simulink model "MCU_PWMPrdChg_Merge"  (R2022b)
settings: Solver=VariableStepAuto  StartTime=0.0  StopTime=10.0  RelTol=1e-3
values from neighbouring files (symbols this model uses):
  C_PWMPrdChg_PwmDefLimit_u16 = 0.0    [MCU_PWMPrdChg_Sldd.sldd]    (also in MCU_PWMPrdChg_Sldd_objects.m = myPackage.Parameter)
  C_PWMPrdChg_PwmHighLimit_u16 = 0.0    [MCU_PWMPrdChg_Sldd.sldd]    (also in MCU_PWMPrdChg_Sldd_objects.m = myPackage.Parameter)
  C_PWMPrdChg_PwmLowLimit_u16 = 0.0    [MCU_PWMPrdChg_Sldd.sldd]    (also in MCU_PWMPrdChg_Sldd_objects.m = myPackage.Parameter)
undefined symbols (not defined in the file or in its folder): MAIN_CPU_FRE, ParamCfg_MotorNp_u16, ParamCfg_PwmFreqHigh_u16, ParamCfg_PwmFreqLow_u16, ParamCfg_PwmLowSpeed_u16, ParamCfg_Pwmprdchgen_u16, ParamCfg_PwmPrdChgEn_u16, ParamCfg_RotateNp_u16, PWM_PERIOD_H
libraries: simulink x2
settings Model: DataDictionary=MCU_PWMPrdChg_Sldd.sldd  Creator=ZYH  LastModifiedBy=ZYH
settings RTWCC: CustomHeaderCode="#include \"myfile.h\""  CustomSource=myfile.c

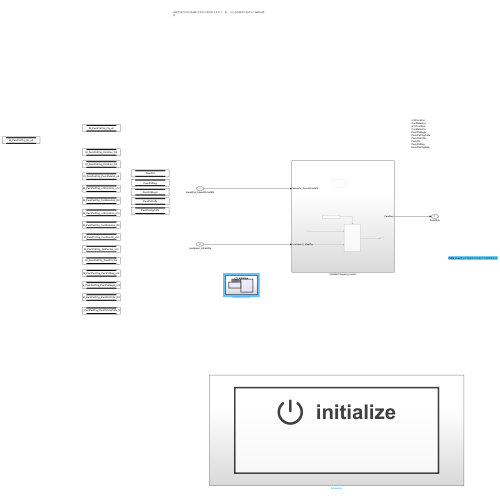
[thumbnail: Simulink's stored preview of the top-level diagram]
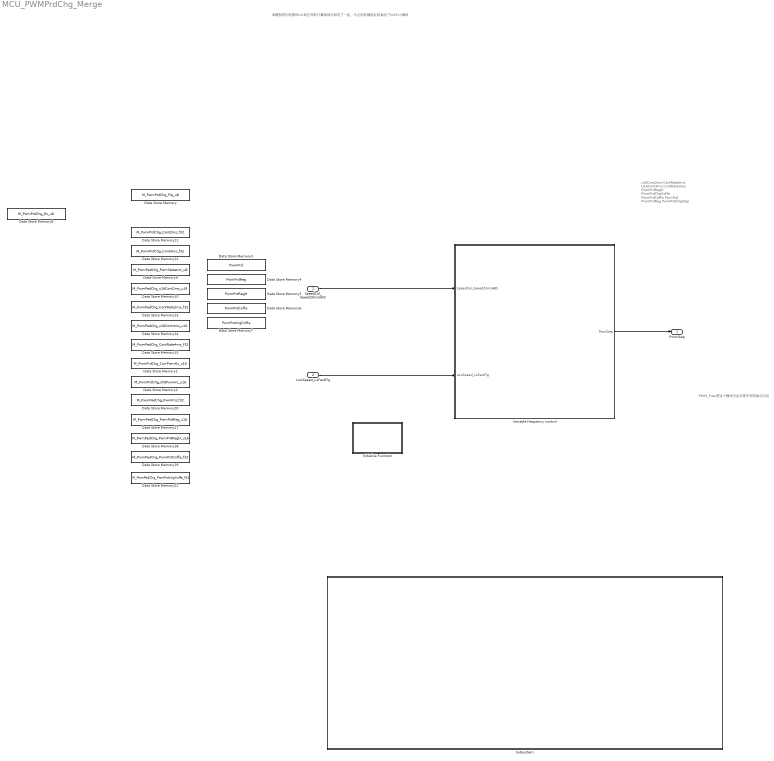
== system MCU_PWMPrdChg_Merge ==
  note: 该模型将代码里的Init和正常的计算两部分和在了一起，与之前的模型比较省去了InitFcn模块
  note: PWM_Freq是这个模块引出还是手写初始化引出
  note: u16Cont2ms
      | ContRate2ms
      | U16Cont4ms
      | ContRate4ms
      | PwmPrdRegH
      | PwmPrdChgCoffe
      | PwmPrdCoffe
      | PwmPrd
      | PwmPrdReg
      | PwmPrdChgStep
  SpeedCal_Speed20msABS : Inport
  LowSpeed_LsFastFlg : Inport  Port=2
  Data Store Memory : DataStoreMemory  DataStoreName=M_PwmPrdChg_Flg_u8  WriteAfterWriteMsg=warning  ShowAdditionalParam=off  OutDataTypeStr=uint8  StateMustResolveToSignalObject=on
  Data Store Memory1 : DataStoreMemory  DataStoreName=M_PwmPrdChg_CurrPwmHz_u16  WriteAfterWriteMsg=warning  ShowAdditionalParam=off  OutDataTypeStr=uint16  StateMustResolveToSignalObject=on
  Data Store Memory10 : DataStoreMemory  DataStoreName=M_PwmPedChg_u16Cont2ms_u16  WriteAfterWriteMsg=warning  ShowAdditionalParam=off  OutDataTypeStr=uint16  StateMustResolveToSignalObject=on
  Data Store Memory11 : DataStoreMemory  DataStoreName=M_PwmPrdChg_Cont2ms_f32  WriteAfterWriteMsg=warning  ShowAdditionalParam=off  OutDataTypeStr=single  StateMustResolveToSignalObject=on
  Data Store Memory12 : DataStoreMemory  DataStoreName=M_PwmPrdChg_Cont4ms_f32  WriteAfterWriteMsg=warning  ShowAdditionalParam=off  OutDataTypeStr=single  StateMustResolveToSignalObject=on
  Data Store Memory13 : DataStoreMemory  DataStoreName=M_PwmPedChg_ContRate2ms_f32  WriteAfterWriteMsg=warning  ShowAdditionalParam=off  OutDataTypeStr=single  StateMustResolveToSignalObject=on
  Data Store Memory14 : DataStoreMemory  DataStoreName=M_PwmPedChg_u16Cont4ms_u16  WriteAfterWriteMsg=warning  ShowAdditionalParam=off  OutDataTypeStr=uint16  StateMustResolveToSignalObject=on
  Data Store Memory15 : DataStoreMemory  DataStoreName=M_PwmPedChg_ContRate4ms_f32  WriteAfterWriteMsg=warning  ShowAdditionalParam=off  OutDataTypeStr=single  StateMustResolveToSignalObject=on
  Data Store Memory17 : DataStoreMemory  DataStoreName=M_PwmPedChg_PwmPrdReg_u16  WriteAfterWriteMsg=warning  ShowAdditionalParam=off  OutDataTypeStr=uint16  StateMustResolveToSignalObject=on
  Data Store Memory18 : DataStoreMemory  DataStoreName=M_PwmPedChg_PwmPrdRegH_u16  WriteAfterWriteMsg=warning  ShowAdditionalParam=off  OutDataTypeStr=uint16  StateMustResolveToSignalObject=on
  Data Store Memory19 : DataStoreMemory  DataStoreName=M_PwmPedChg_PwmPrdCoffe_f32  WriteAfterWriteMsg=warning  ShowAdditionalParam=off  OutDataTypeStr=single  StateMustResolveToSignalObject=on
  Data Store Memory2 : DataStoreMemory  DataStoreName=M_PwmPrdChg_OldPwmHz_u16  WriteAfterWriteMsg=warning  ShowAdditionalParam=off  OutDataTypeStr=uint16  StateMustResolveToSignalObject=on
  Data Store Memory20 : DataStoreMemory  DataStoreName=M_PwmPedChg_PwmPrd_f32  WriteAfterWriteMsg=warning  ShowAdditionalParam=off  OutDataTypeStr=single  StateMustResolveToSignalObject=on
  Data Store Memory21 : DataStoreMemory  DataStoreName=M_PwmPedChg_PwmPrdchgCoffe_f32  WriteAfterWriteMsg=warning  ShowAdditionalParam=off  OutDataTypeStr=single  StateMustResolveToSignalObject=on
  Data Store Memory3 : DataStoreMemory  DataStoreName=PwmPrd  WriteAfterWriteMsg=warning  ShowAdditionalParam=off
  Data Store Memory4 : DataStoreMemory  DataStoreName=PwmPrdReg  WriteAfterWriteMsg=warning  ShowAdditionalParam=off
  Data Store Memory5 : DataStoreMemory  DataStoreName=PwmPrdRegH  WriteAfterWriteMsg=warning  ShowAdditionalParam=off
  Data Store Memory6 : DataStoreMemory  DataStoreName=PwmPrdCoffe  WriteAfterWriteMsg=warning  ShowAdditionalParam=off
  Data Store Memory7 : DataStoreMemory  DataStoreName=PwmPrdchgCoffe  WriteAfterWriteMsg=warning  ShowAdditionalParam=off
  Data Store Memory8 : DataStoreMemory  DataStoreName=M_PwmPrdChg_En_u8  WriteAfterWriteMsg=warning  ShowAdditionalParam=off  OutDataTypeStr=uint8  StateMustResolveToSignalObject=on
  Data Store Memory9 : DataStoreMemory  DataStoreName=M_PwmPedChg_PwmStateInit_u8  WriteAfterWriteMsg=warning  ShowAdditionalParam=off  OutDataTypeStr=uint8  StateMustResolveToSignalObject=on
  Initialize Function : Subsystem  TreatAsAtomicUnit=on
  Subsystem : Subsystem
  Variable frequency control : Subsystem
  PwmStep : Outport
  wires:
  Variable frequency control/1(PwmStep) -> PwmStep/1
  SpeedCal_Speed20msABS/1 -> Variable frequency control/1(SpeedCal_Speed20msABS)
  LowSpeed_LsFastFlg/1 -> Variable frequency control/2(LowSpeed_LsFastFlg)

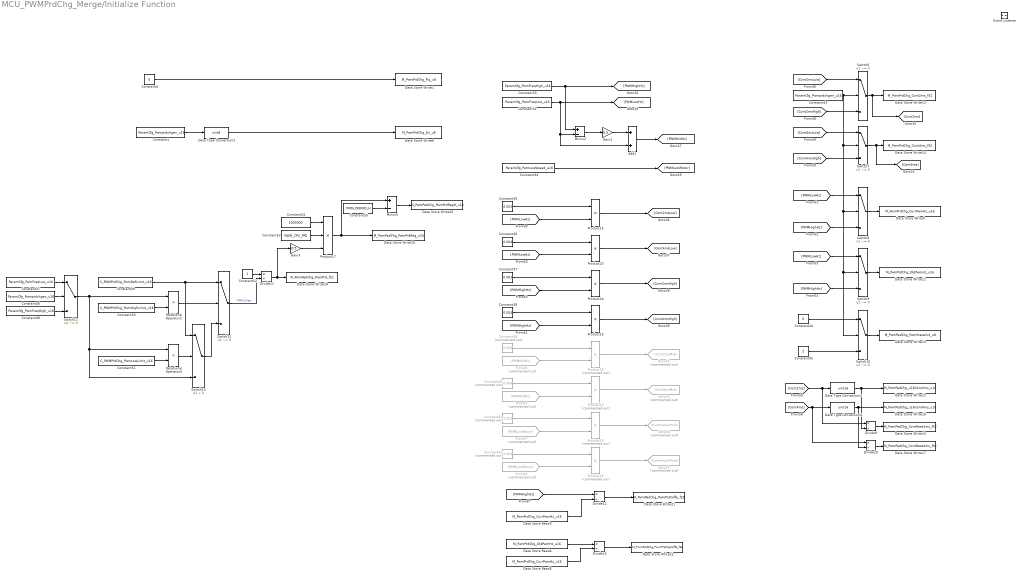
== system MCU_PWMPrdChg_Merge/Initialize Function ==
  Add1 : Sum  OutDataTypeStr=uint16
  Constant1 : Constant  Value=ParamCfg_Pwmprdchgen_u16  OutDataTypeStr=uint16
  Constant32 : Constant  Value=ParamCfg_PwmFreqLow_u16  OutDataTypeStr=uint16
  Constant33 : Constant  Value=ParamCfg_PwmFreqHigh_u16  OutDataTypeStr=uint16
  Constant34 : Constant  Value=ParamCfg_PwmLowSpeed_u16  OutDataTypeStr=uint16
  Constant35 : Constant  Value=0.002  OutDataTypeStr=single
  Constant36 : Constant  Value=0.004  OutDataTypeStr=single
  Constant37 : Constant  Value=0.002  OutDataTypeStr=single
  Constant38 : Constant  Value=0.004  OutDataTypeStr=single
  Constant39 : Constant  Commented=on  Value=0.002  OutDataTypeStr=single
  Constant4 : Constant  Value=0  OutDataTypeStr=uint8
  Constant40 : Constant  Commented=on  Value=0.004  OutDataTypeStr=single
  Constant41 : Constant  Commented=on  Value=0.002  OutDataTypeStr=single
  Constant42 : Constant  Commented=on  Value=0.004  OutDataTypeStr=single
  Constant43 : Constant  Value=ParamCfg_Pwmprdchgen_u16  OutDataTypeStr=uint16
  Constant44 : Constant  Value=0  OutDataTypeStr=uint8
  Constant45 : Constant  Value=2  OutDataTypeStr=uint8
  Constant46 : Constant  Value=ParamCfg_Pwmprdchgen_u16  OutDataTypeStr=uint16
  Constant47 : Constant  Value=ParamCfg_PwmFreqLow_u16  OutDataTypeStr=uint16
  Constant48 : Constant  Value=ParamCfg_PwmFreqHigh_u16  OutDataTypeStr=uint16
  Constant49 : Constant  Value=C_PWMPrdChg_PwmDefLimit_u16  OutDataTypeStr=uint16
  Constant50 : Constant  Value=C_PWMPrdChg_PwmHighLimit_u16  OutDataTypeStr=uint16
  Constant51 : Constant  Value=C_PWMPrdChg_PwmLowLimit_u16  OutDataTypeStr=uint16
  Constant52 : Constant  OutDataTypeStr=single
  Constant53 : Constant  Value=MAIN_CPU_FRE  OutDataTypeStr=uint16
  Constant54 : Constant  Value=1000000  OutDataTypeStr=single
  Constant55 : Constant  Value=PWM_PERIOD_H  OutDataTypeStr=uint16
  Data Store Read3 : DataStoreRead  DataStoreName=M_PwmPrdChg_CurrPwmHz_u16  IndexOptions=Index vector (dialog)  Indices=1  OutputSizes=1
  Data Store Read4 : DataStoreRead  DataStoreName=M_PwmPrdChg_OldPwmHz_u16  IndexOptions=Index vector (dialog)  Indices=1  OutputSizes=1
  Data Store Read5 : DataStoreRead  DataStoreName=M_PwmPrdChg_CurrPwmHz_u16  IndexOptions=Index vector (dialog)  Indices=1  OutputSizes=1
  Data Store Write1 : DataStoreWrite  DataStoreName=M_PwmPrdChg_Flg_u8  IndexOptions=Index vector (dialog)  Indices=1  OutputSizes=1
  Data Store Write10 : DataStoreWrite  DataStoreName=M_PwmPedChg_PwmStateInit_u8  IndexOptions=Index vector (dialog)  Indices=1  OutputSizes=1
  Data Store Write11 : DataStoreWrite  DataStoreName=M_PwmPrdChg_OldPwmHz_u16  IndexOptions=Index vector (dialog)  Indices=1  OutputSizes=1
  Data Store Write12 : DataStoreWrite  DataStoreName=M_PwmPedChg_u16Cont2ms_u16  IndexOptions=Index vector (dialog)  Indices=1  OutputSizes=1
  Data Store Write13 : DataStoreWrite  DataStoreName=M_PwmPrdChg_Cont2ms_f32  IndexOptions=Index vector (dialog)  Indices=1  OutputSizes=1
  Data Store Write14 : DataStoreWrite  DataStoreName=M_PwmPrdChg_Cont4ms_f32  IndexOptions=Index vector (dialog)  Indices=1  OutputSizes=1
  Data Store Write15 : DataStoreWrite  DataStoreName=M_PwmPedChg_ContRate2ms_f32  IndexOptions=Index vector (dialog)  Indices=1  OutputSizes=1
  Data Store Write16 : DataStoreWrite  DataStoreName=M_PwmPedChg_u16Cont4ms_u16  IndexOptions=Index vector (dialog)  Indices=1  OutputSizes=1
  Data Store Write17 : DataStoreWrite  DataStoreName=M_PwmPedChg_ContRate4ms_f32  IndexOptions=Index vector (dialog)  Indices=1  OutputSizes=1
  Data Store Write18 : DataStoreWrite  DataStoreName=M_PwmPedChg_PwmPrd_f32  IndexOptions=Index vector (dialog)  Indices=1  OutputSizes=1
  Data Store Write19 : DataStoreWrite  DataStoreName=M_PwmPedChg_PwmPrdReg_u16  IndexOptions=Index vector (dialog)  Indices=1  OutputSizes=1
  Data Store Write20 : DataStoreWrite  DataStoreName=M_PwmPedChg_PwmPrdRegH_u16  IndexOptions=Index vector (dialog)  Indices=1  OutputSizes=1
  Data Store Write21 : DataStoreWrite  DataStoreName=M_PwmPedChg_PwmPrdCoffe_f32  IndexOptions=Index vector (dialog)  Indices=1  OutputSizes=1
  Data Store Write22 : DataStoreWrite  DataStoreName=M_PwmPedChg_PwmPrdchgCoffe_f32  IndexOptions=Index vector (dialog)  Indices=1  OutputSizes=1
  Data Store Write8 : DataStoreWrite  DataStoreName=M_PwmPrdChg_En_u8  IndexOptions=Index vector (dialog)  Indices=1  OutputSizes=1
  Data Store Write9 : DataStoreWrite  DataStoreName=M_PwmPrdChg_CurrPwmHz_u16  IndexOptions=Index vector (dialog)  Indices=1  OutputSizes=1
  Data Type Conversion2 : DataTypeConversion  OutDataTypeStr=uint8  SaturateOnIntegerOverflow=off  RndMeth=Floor
  Data Type Conversion3 : DataTypeConversion  OutDataTypeStr=uint16  SaturateOnIntegerOverflow=off  RndMeth=Floor
  Data Type Conversion4 : DataTypeConversion  OutDataTypeStr=uint16  SaturateOnIntegerOverflow=off  RndMeth=Floor
  Divide10 : Product  Inputs=*/
  Divide11 : Product  Inputs=*/
  Divide12 : Product  Inputs=*/  OutDataTypeStr=single
  Divide13 : Product  Inputs=*/  OutDataTypeStr=single
  Divide9 : Product  Inputs=*/
  Event Listener : EventListener  DisableCoverage=on  EventName=reset  VariantControl=rtt
  From42 : From  Commented=on  GotoTag=PWMMidHz
  From44 : From  Commented=on  GotoTag=PWMLockRotor
  From45 : From  Commented=on  GotoTag=PWMMidHz
  From47 : From  Commented=on  GotoTag=PWMLockRotor
  Gain2 : Gain  Gain=0.5  ParamDataTypeStr=single  OutDataTypeStr=single
  Gain3 : Gain  Gain=0.5  ParamDataTypeStr=single  OutDataTypeStr=single
  Goto32 : Goto  Commented=on  GotoTag=Cont2msMid
  Goto33 : Goto  Commented=on  GotoTag=Cont4msMid
  Goto34 : Goto  Commented=on  GotoTag=Cont2msLockRotor
  Goto35 : Goto  Commented=on  GotoTag=Cont4msLockRotor
  Minus2 : Sum  Inputs=+-
  Minus3 : Sum  Inputs=+-
  Product{15,23..25} (4 alike) : Product
  Product{16,19..20,26} (4 alike) : Product  Commented=on
  Product17 : Product  Inputs=3  OutDataTypeStr=uint16
  Relational Operator2 : RelationalOperator  Operator=>  OutDataTypeStr=boolean  RndMeth=Simplest  InputSameDT=off
  Relational Operator3 : RelationalOperator  Operator=<  OutDataTypeStr=boolean  RndMeth=Simplest  InputSameDT=off
  Switch{6..12} (7 alike) : Switch  Criteria=u2 ~= 0  SaturateOnIntegerOverflow=off  InputSameDT=off
  Switch13 : Switch  Criteria=u2 > Threshold  SaturateOnIntegerOverflow=off  InputSameDT=off
  wires:
  Constant4/1 -> Data Store Write1/1
  Constant1/1 -> Data Type Conversion2/1
  Data Type Conversion2/1 -> Data Store Write8/1
  Constant33/1 -> Minus2/1, [PWMHighHz]
  Minus2/1 -> Gain2/1
  Gain2/1 -> Add1/1
  Constant32/1 -> Add1/2, Minus2/2, [PWMLowHz]
  Add1/1 -> [PWMMidHz]
  Constant34/1 -> [PWMLockRotor]
  Product15/1 -> [Cont2msLow]
  Constant35/1 -> Product15/1
  [PWMLowHz] -> Product15/2
  Constant36/1 -> Product23/1
  [PWMLowHz] -> Product23/2
  Product23/1 -> [Cont4msLow]
  Constant38/1 -> Product25/1
  Product24/1 -> [Cont2msHigh]
  Product25/1 -> [Cont4msHigh]
  Constant37/1 -> Product24/1
  [PWMHighHz] -> Product24/2
  [PWMHighHz] -> Product25/2
  Product16/1 -> Goto32/1
  Product19/1 -> Goto33/1
  Constant39/1 -> Product16/1
  From42/1 -> Product19/2
  Constant40/1 -> Product19/1
  From45/1 -> Product16/2
  From47/1 -> Product20/2
  Constant42/1 -> Product26/1
  Constant41/1 -> Product20/1
  From44/1 -> Product26/2
  Product26/1 -> Goto35/1
  Product20/1 -> Goto34/1
  Switch7/1 -> [Cont4ms], Data Store Write14/1
  [Cont2msLow] -> Switch6/1
  Switch6/1 -> [Cont2ms], Data Store Write13/1
  [PWMHighHz] -> Switch8/3
  [Cont2msHigh] -> Switch6/3
  [Cont4msHigh] -> Switch7/3
  Switch8/1 -> Data Store Write9/1
  [Cont4msLow] -> Switch7/1
  [PWMLowHz] -> Switch8/1
  [PWMLowHz] -> Switch9/1
  [PWMHighHz] -> Switch9/3
  Switch9/1 -> Data Store Write11/1
  Constant43/1 -> Switch6/2, Switch7/2, Switch8/2, Switch10/2, Switch9/2
  Switch10/1 -> Data Store Write10/1
  Constant44/1 -> Switch10/1
  Constant45/1 -> Switch10/3
  [Cont2ms] -> Divide9/1, Data Type Conversion3/1
  [Cont4ms] -> Divide10/1, Data Type Conversion4/1
  Data Type Conversion4/1 -> Divide10/2, Data Store Write16/1
  Data Type Conversion3/1 -> Divide9/2, Data Store Write12/1
  Divide9/1 -> Data Store Write15/1
  Divide10/1 -> Data Store Write17/1
  Constant51/1 -> Relational Operator3/2
  Switch13/1 -> Switch12/3
  Constant46/1 -> Switch11/2
  Constant54/1 -> Product17/1
  Constant52/1 -> Divide11/1
  Divide11/1 -> Data Store Write18/1, Gain3/1
  Gain3/1 -> Product17/3
  Constant50/1 -> Relational Operator2/2
  Relational Operator2/1 -> Switch12/2
  Constant47/1 -> Switch11/1
  Constant49/1 -> Switch12/1, Switch13/1
  Constant55/1 -> Minus3/2
  Switch12/1 -> Divide11/2  "PWM_Freq"
  Switch11/1 -> Relational Operator2/1, Relational Operator3/1, Switch13/3
  Constant48/1 -> Switch11/3
  Relational Operator3/1 -> Switch13/2
  Constant53/1 -> Product17/2
  Product17/1 -> Minus3/1, Data Store Write19/1
  Minus3/1 -> Data Store Write20/1
  Data Store Read3/1 -> Divide12/2
  Divide13/1 -> Data Store Write22/1
  Divide12/1 -> Data Store Write21/1
  [PWMHighHz] -> Divide12/1
  Data Store Read4/1 -> Divide13/1
  Data Store Read5/1 -> Divide13/2

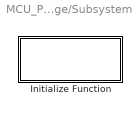
== system MCU_PWMPrdChg_Merge/Subsystem ==
  Initialize Function : Subsystem  TreatAsAtomicUnit=on

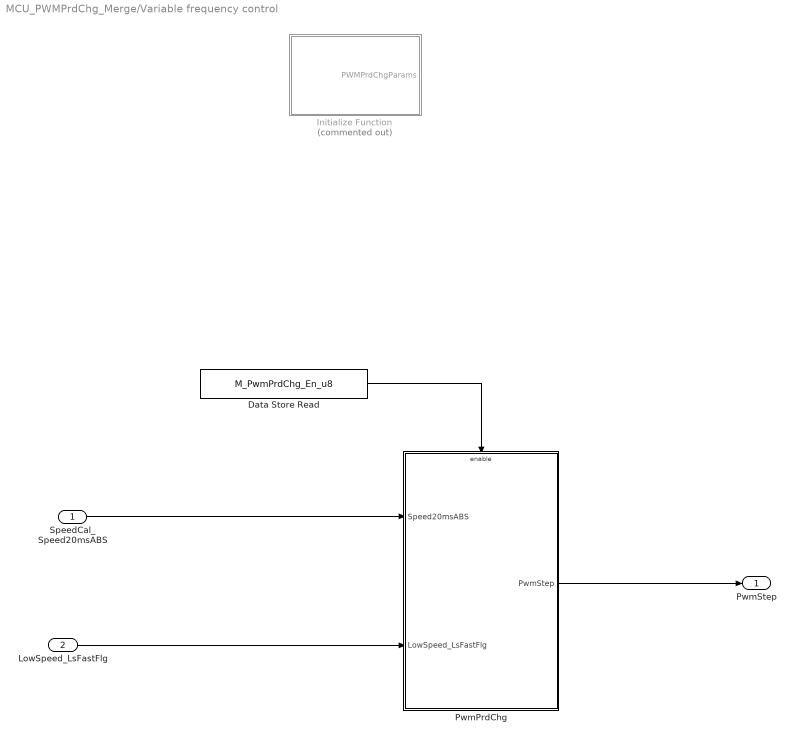
== system MCU_PWMPrdChg_Merge/Variable frequency control ==
  SpeedCal_Speed20msABS : Inport
  LowSpeed_LsFastFlg : Inport  Port=2
  Data Store Read : DataStoreRead  DataStoreName=M_PwmPrdChg_En_u8  IndexOptions=Index vector (dialog)  Indices=1  OutputSizes=1
  Initialize Function : Subsystem  Commented=on  TreatAsAtomicUnit=on
  PwmPrdChg : Subsystem
  PwmStep : Outport
  wires:
  SpeedCal_Speed20msABS/1 -> PwmPrdChg/1(Speed20msABS)
  LowSpeed_LsFastFlg/1 -> PwmPrdChg/2(LowSpeed_LsFastFlg)
  Data Store Read/1 -> PwmPrdChg/Enable
  PwmPrdChg/1(PwmStep) -> PwmStep/1

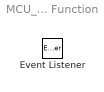
== system MCU_PWMPrdChg_Merge/Subsystem/Initialize Function ==
  Event Listener : EventListener  DisableCoverage=on  EventName=reset

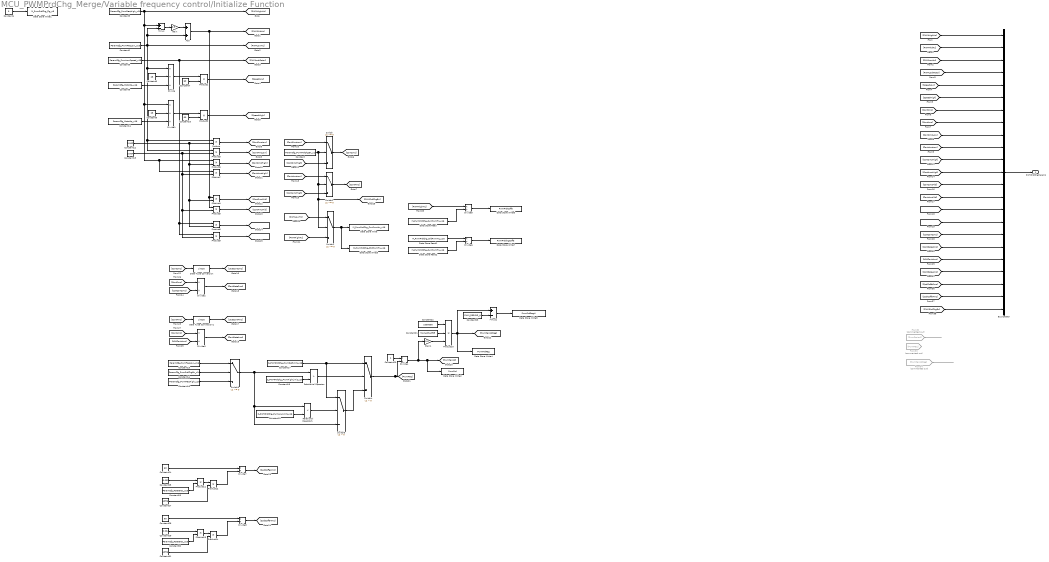
== system MCU_PWMPrdChg_Merge/Variable frequency control/Initialize Function ==
  Add : Sum  OutDataTypeStr=uint16
  Bus Creator : BusCreator  Inputs=23  OutDataTypeStr=Bus: PwmPrdChgBus  NonVirtualBus=on
  Constant : Constant  Value=ParamCfg_PwmPrdChgEn_u16  OutDataTypeStr=uint16
  Constant{7,10,24,28} (4 alike) : Constant  Value=60  OutDataTypeStr=single
  Constant11 : Constant  Value=ParamCfg_MotorNp_u16  OutDataTypeStr=uint16
  Constant12 : Constant  Value=0.002  OutDataTypeStr=single
  Constant13 : Constant  Value=0.004  OutDataTypeStr=single
  Constant14 : Constant  Value=ParamCfg_PwmPrdChgEn_u16  OutDataTypeStr=uint16
  Constant15 : Constant  Value=ParamCfg_PwmFreqLow_u16  OutDataTypeStr=uint16
  Constant16 : Constant  Value=ParamCfg_PwmFreqHigh_u16  OutDataTypeStr=uint16
  Constant17 : Constant  Value=C_PWMPrdChg_PwmDefLimit_u16  OutDataTypeStr=uint16
  Constant18 : Constant  Value=C_PWMPrdChg_PwmHighLimit_u16  OutDataTypeStr=uint16
  Constant19 : Constant  Value=C_PWMPrdChg_PwmLowLimit_u16  OutDataTypeStr=uint16
  Constant2 : Constant  Value=ParamCfg_PwmFreqLow_u16  OutDataTypeStr=uint16
  Constant20 : Constant  OutDataTypeStr=single
  Constant21 : Constant  Value=MAIN_CPU_FRE  OutDataTypeStr=uint16
  Constant22 : Constant  Value=1000000  OutDataTypeStr=single
  Constant23 : Constant  Value=PWM_PERIOD_H  OutDataTypeStr=uint16
  Constant25 : Constant  Value=0.002  OutDataTypeStr=single
  Constant26 : Constant  Value=ParamCfg_RotateNp_u16  OutDataTypeStr=uint16
  Constant27 : Constant  Value=4096  OutDataTypeStr=single
  Constant29 : Constant  Value=0.004  OutDataTypeStr=single
  Constant3 : Constant  Value=ParamCfg_PwmFreqHigh_u16  OutDataTypeStr=uint16
  Constant30 : Constant  Value=ParamCfg_RotateNp_u16  OutDataTypeStr=uint16
  Constant31 : Constant  Value=4096  OutDataTypeStr=single
  Constant4 : Constant  Value=0  OutDataTypeStr=uint8
  Constant5 : Constant  Value=ParamCfg_PwmLowSpeed_u16  OutDataTypeStr=uint16
  Constant6 : Constant  Value=25  OutDataTypeStr=single
  Constant8 : Constant  Value=ParamCfg_MotorNp_u16  OutDataTypeStr=uint16
  Constant9 : Constant  Value=25  OutDataTypeStr=single
  Data Store Read : DataStoreRead  DataStoreName=M_PwmPrdChg_CurrPwmHz_u16  IndexOptions=Index vector (dialog)  Indices=1  OutputSizes=1
  Data Store Read1 : DataStoreRead  DataStoreName=M_PwmPrdChg_OldPwmHz_u16  IndexOptions=Index vector (dialog)  Indices=1  OutputSizes=1
  Data Store Read2 : DataStoreRead  DataStoreName=M_PwmPrdChg_CurrPwmHz_u16  IndexOptions=Index vector (dialog)  Indices=1  OutputSizes=1
  Data Store Write : DataStoreWrite  DataStoreName=M_PwmPrdChg_CurrPwmHz_u16  IndexOptions=Index vector (dialog)  Indices=1  OutputSizes=1
  Data Store Write1 : DataStoreWrite  DataStoreName=M_PwmPrdChg_Flg_u8  IndexOptions=Index vector (dialog)  Indices=1  OutputSizes=1
  Data Store Write2 : DataStoreWrite  DataStoreName=PwmPrd  IndexOptions=Index vector (dialog)  Indices=1  OutputSizes=1
  Data Store Write3 : DataStoreWrite  DataStoreName=M_PwmPrdChg_OldPwmHz_u16  IndexOptions=Index vector (dialog)  Indices=1  OutputSizes=1
  Data Store Write4 : DataStoreWrite  DataStoreName=PwmPrdReg  IndexOptions=Index vector (dialog)  Indices=1  OutputSizes=1
  Data Store Write5 : DataStoreWrite  DataStoreName=PwmPrdRegH  IndexOptions=Index vector (dialog)  Indices=1  OutputSizes=1
  Data Store Write6 : DataStoreWrite  DataStoreName=PwmPrdCoffe  IndexOptions=Index vector (dialog)  Indices=1  OutputSizes=1
  Data Store Write7 : DataStoreWrite  DataStoreName=PwmPrdchgCoffe  IndexOptions=Index vector (dialog)  Indices=1  OutputSizes=1
  Data Type Conversion : DataTypeConversion  OutDataTypeStr=uint16  SaturateOnIntegerOverflow=off  RndMeth=Floor
  Data Type Conversion1 : DataTypeConversion  OutDataTypeStr=uint16  SaturateOnIntegerOverflow=off  RndMeth=Floor
  Divide : Product  Inputs=*//
  Divide1 : Product  Inputs=*//
  Divide{2..4,7..8} (5 alike) : Product  Inputs=*/
  Divide5 : Product  Inputs=*/  OutDataTypeStr=single
  Divide6 : Product  Inputs=*/  OutDataTypeStr=single
  From32 : From  Commented=on  GotoTag=PwmPeriod
  From33 : From  Commented=on  GotoTag=PwmFreq
  From34 : From  Commented=on  GotoTag=PwmPeriodReg
  Gain : Gain  Gain=0.5  ParamDataTypeStr=single  OutDataTypeStr=single
  Gain1 : Gain  Gain=0.5  ParamDataTypeStr=single  OutDataTypeStr=single
  Minus : Sum  Inputs=+-
  Minus1 : Sum  Inputs=+-
  Product{,1..9,11..14} (14 alike) : Product
  Product10 : Product  Inputs=3  OutDataTypeStr=uint16
  Relational Operator : RelationalOperator  Operator=>  OutDataTypeStr=boolean  RndMeth=Simplest  InputSameDT=off
  Relational Operator1 : RelationalOperator  Operator=<  OutDataTypeStr=boolean  RndMeth=Simplest  InputSameDT=off
  Switch{,1..3} (4 alike) : Switch  Criteria=u2 ~= 0  SaturateOnIntegerOverflow=off  InputSameDT=off
  Switch4 : Switch  Criteria=u2 > Threshold  SaturateOnIntegerOverflow=off  InputSameDT=off
  Switch5 : Switch  Criteria=u2 > Threshold  SaturateOnIntegerOverflow=off  InputSameDT=off
  PWMPrdChgParams : Outport
  wires:
  Gain/1 -> Add/1
  Minus/1 -> Gain/1
  Constant2/1 -> Product3/1, Product/1, Divide/1, [PWMLowHz], Add/2, Minus/2
  Constant3/1 -> Product7/1, Product6/1, Divide1/1, Minus/1, [PWMHighHz]
  Constant4/1 -> Data Store Write1/1
  Bus Creator/1 -> PWMPrdChgParams/1
  Add/1 -> [PWMMidHz], Product5/1, Product4/1
  Constant5/1 -> [PWMLockRotor], Product9/1, Product8/1
  Constant6/1 -> Divide/2
  Divide/1 -> Product1/1
  Constant7/1 -> Product1/2
  Constant8/1 -> Divide/3
  Product1/1 -> [SpeedLow]
  Divide1/1 -> Product2/1
  Constant10/1 -> Product2/2
  Constant11/1 -> Divide1/3
  Constant9/1 -> Divide1/2
  Product2/1 -> [SpeedHigh]
  Constant12/1 -> Product4/2, Product8/2, Product6/2, Product/2
  Constant13/1 -> Product5/2, Product9/2, Product7/2, Product3/2
  Product/1 -> [Cont2msLow]
  Product3/1 -> [Cont4msLow]
  Product4/1 -> [Cont2msMid]
  Product5/1 -> [Cont4msMid]
  Product6/1 -> [Cont2msHigh]
  Product7/1 -> [Cont4msHigh]
  Product8/1 -> [Cont2msLockRotor]  "Cont2msLockRotor"
  Product9/1 -> [Cont4msLockRotor]
  Constant/1 -> Switch2/2, [PWMPrdChgEn], Switch1/2, Switch/2
  [PWMHighHz] -> Bus Creator/1  "PWMHighHz"
  [PWMMidHz] -> Bus Creator/2  "PWMMidHz"
  [PWMLowHz] -> Bus Creator/3  "PWMLowHz"
  [PWMLockRotor] -> Bus Creator/4  "PWMLockRotor"
  [SpeedLow] -> Bus Creator/5  "SpeedLow"
  [SpeedHigh] -> Bus Creator/6  "SpeedHigh"
  Switch/1 -> [Cont2ms]
  [Cont2ms] -> Bus Creator/7  "Cont2ms"
  Switch1/1 -> [Cont4ms]
  [Cont4ms] -> Bus Creator/8  "Cont4ms"
  [Cont2msLow] -> Bus Creator/9  "Cont2msLow"
  [Cont4msLow] -> Bus Creator/10  "Cont4msLow"
  [Cont2msLow] -> Switch/1
  [Cont2msHigh] -> Bus Creator/11  "Cont2msHigh"
  [Cont2msHigh] -> Switch/3
  [Cont4msLow] -> Switch1/1
  [Cont4msHigh] -> Bus Creator/12  "Cont4msHigh"
  [Cont4msHigh] -> Switch1/3
  [Cont2msMid] -> Bus Creator/13  "Cont2msMid"
  [Cont4msMid] -> Bus Creator/14  "Cont4msMid"
  [Cont2msLockRotor] -> Bus Creator/15  "Cont2msLockRotor"
  [Cont4msLockRotor] -> Bus Creator/16  "Cont4msLockRotor"
  [PWMLowHz] -> Switch2/1
  Switch2/1 -> Data Store Write3/1, Data Store Write/1
  [PWMHighHz] -> Switch2/3
  [Cont2ms] -> Data Type Conversion/1
  Data Type Conversion/1 -> [U16Cont2ms]
  [Cont4ms] -> Data Type Conversion1/1
  Data Type Conversion1/1 -> [U16Cont4ms]
  [Cont2ms] -> Divide2/1
  [U16Cont2ms] -> Divide2/2
  [Cont4ms] -> Divide3/1
  [U16Cont4ms] -> Divide3/2
  Divide2/1 -> [ContRate2ms]
  Divide3/1 -> [ContRate4ms]
  [U16Cont2ms] -> Bus Creator/17  "U16Cont2ms"
  [ContRate2ms] -> Bus Creator/18  "ContRate2ms"
  [U16Cont4ms] -> Bus Creator/19  "U16Cont4ms"
  [ContRate4ms] -> Bus Creator/20  "ContRate4ms"
  Switch5/1 -> Switch4/3
  Relational Operator1/1 -> Switch5/2
  Constant19/1 -> Relational Operator1/2
  Relational Operator/1 -> Switch4/2
  Constant14/1 -> Switch3/2
  Constant16/1 -> Switch3/3
  Switch3/1 -> Switch5/3, Relational Operator1/1, Relational Operator/1
  Constant18/1 -> Relational Operator/2
  Constant17/1 -> Switch5/1, Switch4/1
  Constant15/1 -> Switch3/1
  Switch4/1 -> [PwmFreq], Divide4/2
  From32/1 -> ?  "PwmPeriod"
  Constant20/1 -> Divide4/1
  Divide4/1 -> Gain1/1, Data Store Write2/1, [PwmPeriod]
  Gain1/1 -> Product10/3
  Constant21/1 -> Product10/2
  Constant22/1 -> Product10/1
  Product10/1 -> Minus1/1, Data Store Write4/1, [PwmPeriodReg]
  From34/1 -> ?  "PwmPeriodReg"
  Constant23/1 -> Minus1/2
  Minus1/1 -> Data Store Write5/1
  [PWMHighHz] -> Divide5/1
  Data Store Read/1 -> Divide5/2
  Divide5/1 -> Data Store Write6/1
  Data Store Read1/1 -> Divide6/1
  Data Store Read2/1 -> Divide6/2
  Divide6/1 -> Data Store Write7/1
  Constant24/1 -> Divide7/1
  Constant25/1 -> Product11/1
  Constant26/1 -> Product11/2
  Product11/1 -> Product12/1
  Constant27/1 -> Product12/2
  Product12/1 -> Divide7/2
  Divide7/1 -> [SpdCoffe2ms]
  [SpdCoffe2ms] -> Bus Creator/21  "SpdCoffe2ms"
  Constant29/1 -> Product13/1
  Constant31/1 -> Product14/2
  Constant28/1 -> Divide8/1
  Product14/1 -> Divide8/2
  Constant30/1 -> Product13/2
  Product13/1 -> Product14/1
  Divide8/1 -> [SpdCoffe4ms]
  [SpdCoffe4ms] -> Bus Creator/22  "SpdCoffe4ms"
  [PWMPrdChgEn] -> Bus Creator/23  "PWMPrdChgEn"

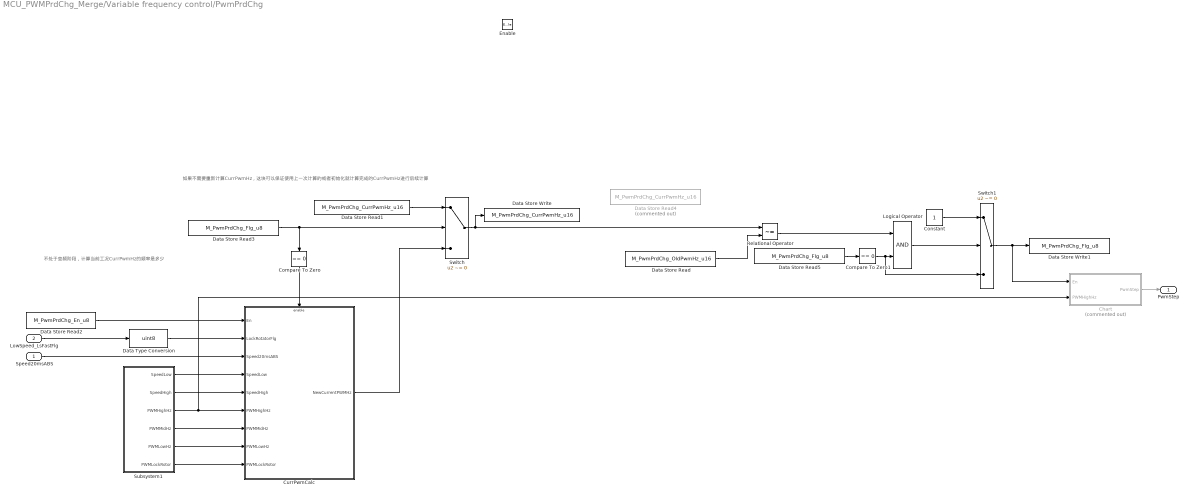
== system MCU_PWMPrdChg_Merge/Variable frequency control/PwmPrdChg ==
  note: 不处于变频阶段，计算当前工况CurrPwmHz的频率是多少
  note: 如果不需要重新计算CurrPwmHz，这块可以保证使用上一次计算的或者初始化就计算完成的CurrPwmHz进行后续计算
  Speed20msABS : Inport
  LowSpeed_LsFastFlg : Inport  Port=2
  Enable : EnablePort
  Chart : Stateflow chart  Commented=on  TreatAsAtomicUnit=on
  Compare To Zero : simulink/Logic and Bit Operations/Compare To Zero  relop===  OutDataTypeStr=boolean
  Compare To Zero1 : simulink/Logic and Bit Operations/Compare To Zero  relop===  OutDataTypeStr=boolean
  Constant : Constant  OutDataTypeStr=uint8
  CurrPwmCalc : Subsystem
  Data Store Read : DataStoreRead  DataStoreName=M_PwmPrdChg_OldPwmHz_u16  IndexOptions=Index vector (dialog)  Indices=1  OutputSizes=1
  Data Store Read1 : DataStoreRead  DataStoreName=M_PwmPrdChg_CurrPwmHz_u16  IndexOptions=Index vector (dialog)  Indices=1  OutputSizes=1
  Data Store Read2 : DataStoreRead  DataStoreName=M_PwmPrdChg_En_u8  IndexOptions=Index vector (dialog)  Indices=1  OutputSizes=1
  Data Store Read3 : DataStoreRead  DataStoreName=M_PwmPrdChg_Flg_u8  IndexOptions=Index vector (dialog)  Indices=1  OutputSizes=1
  Data Store Read4 : DataStoreRead  Commented=on  DataStoreName=M_PwmPrdChg_CurrPwmHz_u16  IndexOptions=Index vector (dialog)  Indices=1  OutputSizes=1
  Data Store Read5 : DataStoreRead  DataStoreName=M_PwmPrdChg_Flg_u8  IndexOptions=Index vector (dialog)  Indices=1  OutputSizes=1
  Data Store Write : DataStoreWrite  DataStoreName=M_PwmPrdChg_CurrPwmHz_u16  IndexOptions=Index vector (dialog)  Indices=1  OutputSizes=1
  Data Store Write1 : DataStoreWrite  DataStoreName=M_PwmPrdChg_Flg_u8  IndexOptions=Index vector (dialog)  Indices=1  OutputSizes=1
  Data Type Conversion : DataTypeConversion  OutDataTypeStr=uint8  SaturateOnIntegerOverflow=off  RndMeth=Floor
  Logical Operator : Logic  AllPortsSameDT=off  OutDataTypeStr=boolean
  Relational Operator : RelationalOperator  Operator=~=  OutDataTypeStr=boolean  RndMeth=Simplest  InputSameDT=off
  Subsystem1 : Subsystem
  Switch : Switch  Criteria=u2 ~= 0  SaturateOnIntegerOverflow=off  InputSameDT=off
  Switch1 : Switch  Criteria=u2 ~= 0  SaturateOnIntegerOverflow=off  InputSameDT=off
  PwmStep : Outport
  wires:
  Data Store Read1/1 -> Switch/1
  CurrPwmCalc/1(NewCurrentPWMHz) -> Switch/3
  Data Store Read/1 -> Relational Operator/2
  LowSpeed_LsFastFlg/1 -> Data Type Conversion/1
  Data Type Conversion/1 -> CurrPwmCalc/2(LockRotatorFlg)
  Speed20msABS/1 -> CurrPwmCalc/3(Speed20msABS)
  Subsystem1/1(SpeedLow) -> CurrPwmCalc/4(SpeedLow)
  Subsystem1/2(SpeedHigh) -> CurrPwmCalc/5(SpeedHigh)
  Subsystem1/3(PWMHighHz) -> Chart/2(PWMHighHz), CurrPwmCalc/6(PWMHighHz)
  Subsystem1/4(PWMMidHz) -> CurrPwmCalc/7(PWMMidHz)
  Subsystem1/5(PWMLowHz) -> CurrPwmCalc/8(PWMLowHz)
  Subsystem1/6(PWMLockRotor) -> CurrPwmCalc/9(PWMLockRotor)
  Data Store Read2/1 -> CurrPwmCalc/1(En)
  Switch/1 -> Relational Operator/1, Data Store Write/1
  Data Store Read3/1 -> Compare To Zero/1, Switch/2
  Relational Operator/1 -> Logical Operator/1
  Compare To Zero/1 -> CurrPwmCalc/Enable
  Logical Operator/1 -> Switch1/2
  Constant/1 -> Switch1/1
  Data Store Read5/1 -> Compare To Zero1/1
  Switch1/1 -> Chart/1(En), Data Store Write1/1
  Chart/1(PwmStep) -> PwmStep/1
  Compare To Zero1/1 -> Switch1/3, Logical Operator/2

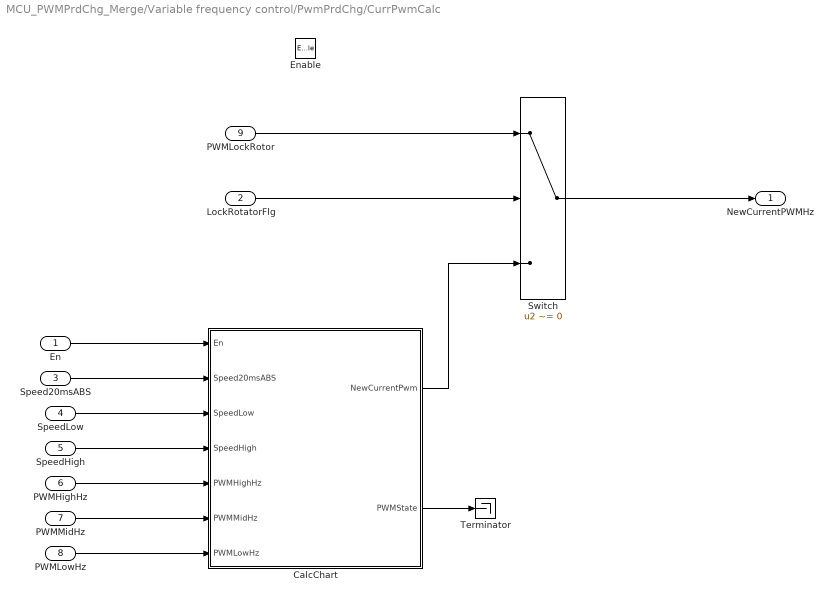
== system MCU_PWMPrdChg_Merge/Variable frequency control/PwmPrdChg/CurrPwmCalc ==
  En : Inport
  LockRotatorFlg : Inport  Port=2
  Speed20msABS : Inport  Port=3
  SpeedLow : Inport  Port=4
  SpeedHigh : Inport  Port=5
  PWMHighHz : Inport  Port=6
  PWMMidHz : Inport  Port=7
  PWMLowHz : Inport  Port=8
  PWMLockRotor : Inport  Port=9
  Enable : EnablePort
  CalcChart : Stateflow chart  TreatAsAtomicUnit=on
  Switch : Switch  Criteria=u2 ~= 0  SaturateOnIntegerOverflow=off  InputSameDT=off
  Terminator : Terminator
  NewCurrentPWMHz : Outport
  wires:
  LockRotatorFlg/1 -> Switch/2
  PWMLockRotor/1 -> Switch/1
  En/1 -> CalcChart/1(En)
  Speed20msABS/1 -> CalcChart/2(Speed20msABS)
  SpeedLow/1 -> CalcChart/3(SpeedLow)
  SpeedHigh/1 -> CalcChart/4(SpeedHigh)
  PWMHighHz/1 -> CalcChart/5(PWMHighHz)
  PWMMidHz/1 -> CalcChart/6(PWMMidHz)
  PWMLowHz/1 -> CalcChart/7(PWMLowHz)
  CalcChart/2(PWMState) -> Terminator/1
  CalcChart/1(NewCurrentPwm) -> Switch/3
  Switch/1 -> NewCurrentPWMHz/1

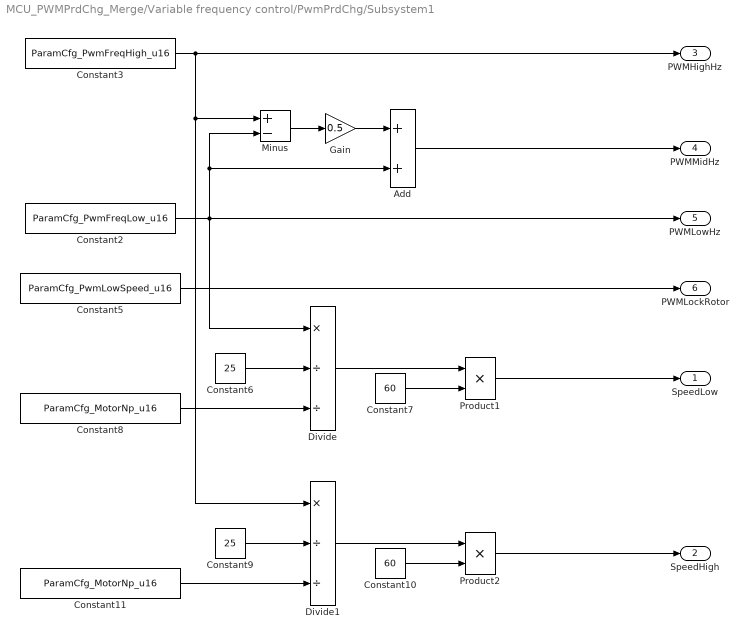
== system MCU_PWMPrdChg_Merge/Variable frequency control/PwmPrdChg/Subsystem1 ==
  Add : Sum  OutDataTypeStr=uint16
  Constant10 : Constant  Value=60  OutDataTypeStr=single
  Constant11 : Constant  Value=ParamCfg_MotorNp_u16  OutDataTypeStr=uint16
  Constant2 : Constant  Value=ParamCfg_PwmFreqLow_u16  OutDataTypeStr=uint16
  Constant3 : Constant  Value=ParamCfg_PwmFreqHigh_u16  OutDataTypeStr=uint16
  Constant5 : Constant  Value=ParamCfg_PwmLowSpeed_u16  OutDataTypeStr=uint16
  Constant6 : Constant  Value=25  OutDataTypeStr=single
  Constant7 : Constant  Value=60  OutDataTypeStr=single
  Constant8 : Constant  Value=ParamCfg_MotorNp_u16  OutDataTypeStr=uint16
  Constant9 : Constant  Value=25  OutDataTypeStr=single
  Divide : Product  Inputs=*//
  Divide1 : Product  Inputs=*//
  Gain : Gain  Gain=0.5  ParamDataTypeStr=single  OutDataTypeStr=single
  Minus : Sum  Inputs=+-
  Product1 : Product
  Product2 : Product
  SpeedLow : Outport
  SpeedHigh : Outport  Port=2
  PWMHighHz : Outport  Port=3
  PWMMidHz : Outport  Port=4
  PWMLowHz : Outport  Port=5
  PWMLockRotor : Outport  Port=6
  wires:
  Constant3/1 -> PWMHighHz/1, Divide1/1, Minus/1
  Product2/1 -> SpeedHigh/1
  Constant6/1 -> Divide/2
  Constant10/1 -> Product2/2
  Gain/1 -> Add/1
  Constant7/1 -> Product1/2
  Divide/1 -> Product1/1
  Minus/1 -> Gain/1
  Constant11/1 -> Divide1/3
  Divide1/1 -> Product2/1
  Constant2/1 -> PWMLowHz/1, Divide/1, Add/2, Minus/2
  Constant5/1 -> PWMLockRotor/1
  Product1/1 -> SpeedLow/1
  Add/1 -> PWMMidHz/1
  Constant8/1 -> Divide/3
  Constant9/1 -> Divide1/2

== stateflow chart MCU_PWMPrdChg_Merge/Variable frequency control/PwmPrdChg/Chart ==
  note: Do not put any code along
      | the transitions that run
      | down the right side!
  (default) -> (junction 2)
  (junction 2) -> (junction 4) : [En == true]{PwmStep = PwmStep+1}
  (junction 4) -> (junction 6) [order 1] : [PwmStep >4]{PwmStep =0;M_PwmPrdChg_Flg_u8 = false;M_PwmPrdChg_OldPwmHz_u16 = M_PwmPrdChg_CurrPwmHz_u16}
  (junction 4) -> (junction 6) [order 2]
  (junction 6) -> (junction 33)
  (junction 33) -> (junction 34) [order 1] : [PwmStep == 1]
  (junction 33) -> (junction 37) [order 2]
  (junction 34) -> (junction 35)
  (junction 35) -> (junction 36)
  (junction 36) -> (junction 40)
  (junction 37) -> (junction 38) [order 1] : [PwmStep == 2]
  (junction 37) -> (junction 41) [order 2]
  (junction 38) -> (junction 39) : {
      | M_PwmPedChg_PwmPrd_f32 = M_PwmPrdChg_CurrPwmHz_u16
      | M_PwmPedChg_PwmPrdReg_u16 = M_PwmPedChg_PwmPrd_f32 * 0.5*MAIN_CPU_FRE*1000000
      | PWMOutputPhasePrd(M_PwmPedChg_PwmPrdReg_u16)
      | }
  (junction 39) -> (junction 40)
  (junction 40) -> (junction 44)
  (junction 41) -> (junction 42) [order 1] : [PwmStep == 3]
  (junction 41) -> (junction 45) [order 2]
  (junction 42) -> (junction 43) : {
      | M_PwmPedChg_PwmPrdCoffe_f32=PWMHighHz/M_PwmPrdChg_CurrPwmHz_u16
      | M_PwmPedChg_PwmPrdchgCoffe_f32 = M_PwmPrdChg_OldPwmHz_u16/M_PwmPrdChg_CurrPwmHz_u16
      | M_PwmPedChg_PwmPrdRegH_u16 = M_PwmPedChg_PwmPrdReg_u16 - PWM_PERIOD_H
      | }
  (junction 43) -> (junction 44)
  (junction 44) -> (junction 48)
  (junction 45) -> (junction 46) [order 1] : [PwmStep == 4]
  (junction 45) -> (junction 49) [order 2]
  (junction 46) -> (junction 47) : {
      | M_PwmPrdChg_Cont2ms_f32 = 0.002*M_PwmPrdChg_CurrPwmHz_u16
      | M_PwmPrdChg_Cont4ms_f32 = 0.004 *M_PwmPrdChg_CurrPwmHz_u16
      | M_PwmPedChg_u16Cont2ms_u16 = uint16(M_PwmPrdChg_Cont2ms_f32)
      | M_PwmPedChg_ContRate2ms_f32 = M_PwmPrdChg_Cont2ms_f32/M_PwmPedChg_u16Cont2ms_u16
      | M_PwmPedChg_u16Cont4ms_u16=uint16(M_PwmPrdChg_Cont4ms_f32)
      | M_PwmPedChg_ContRate4ms_f32 = M_PwmPrdChg_Cont4ms_f32/M_PwmPedChg_u16Cont4ms_u16
      | }
  (junction 47) -> (junction 48)
  (junction 48) -> (junction 50)
  (junction 50) -> (junction 49)
  (junction 49) -> (junction 51)
  data: En input uint8; PwmStep output uint8 =0; M_PwmPedChg_PwmPrd_f32 data_store_memory; M_PwmPrdChg_CurrPwmHz_u16 data_store_memory; MAIN_CPU_FRE parameter; M_PwmPedChg_PwmPrdReg_u16 data_store_memory; PWMHighHz input; M_PwmPedChg_PwmPrdCoffe_f32 data_store_memory; M_PwmPedChg_PwmPrdchgCoffe_f32 data_store_memory; M_PwmPrdChg_OldPwmHz_u16 data_store_memory; M_PwmPedChg_PwmPrdRegH_u16 data_store_memory; PWM_PERIOD_H parameter; M_PwmPrdChg_Cont4ms_f32 data_store_memory; M_PwmPrdChg_Cont2ms_f32 data_store_memory; M_PwmPedChg_u16Cont2ms_u16 data_store_memory; M_PwmPedChg_ContRate2ms_f32 data_store_memory; M_PwmPedChg_u16Cont4ms_u16 data_store_memory; M_PwmPedChg_ContRate4ms_f32 data_store_memory; M_PwmPrdChg_Flg_u8 data_store_memory

== stateflow chart MCU_PWMPrdChg_Merge/Variable frequency control/PwmPrdChg/CurrPwmCalc/CalcChart ==
  state Init
  state STATE_LOW
    PWMState = Low;
    NewCurrentPwm = PWMLowHz;
  state STATE_HIGH
    PWMState = High;
    NewCurrentPwm = PWMHighHz;
  state STATE_MID
    PWMState = Mid;
    NewCurrentPwm = PWMMidHz;
  (default) -> Init
  Init -> (junction 5)
  (junction 5) -> STATE_LOW [order 2] : [En == true]
  (junction 5) -> STATE_HIGH [order 1] : [En == false]
  STATE_LOW -> STATE_MID : [Speed20msABS>SpeedLow]
  STATE_MID -> STATE_HIGH [order 1] : [Speed20msABS>SpeedHigh]
  STATE_HIGH -> STATE_MID : [Speed20msABS < SpeedHigh-SpeedLimit]
  STATE_MID -> STATE_LOW [order 2] : [Speed20msABS < SpeedLow-SpeedLimit]
  data: En input; Speed20msABS input single; SpeedLow input; SpeedHigh input; PWMHighHz input; PWMMidHz input; PWMLowHz input; Low constant uint8 =0; NewCurrentPwm output uint16; PWMState output double; Mid constant uint8 =1; High constant uint8 =2; SpeedLimit constant single
